simulink model "block6_simulink"  (R2025a)
settings: Solver=ode23tb  StartTime=0.0  StopTime=9  RelTol=1e-3
values from neighbouring files (symbols this model uses):
  K = inv(Rm) * B' * P    [block_6.m]
undefined symbols (not defined in the file or in its folder): G, I0_nom, iL_nom, Jac_A_lin, Jac_B_lin, R, V0, vC_nom
libraries: SignalEditorBlockLib x1
settings Model: Creator=arntzen  LastModifiedBy=arntzen

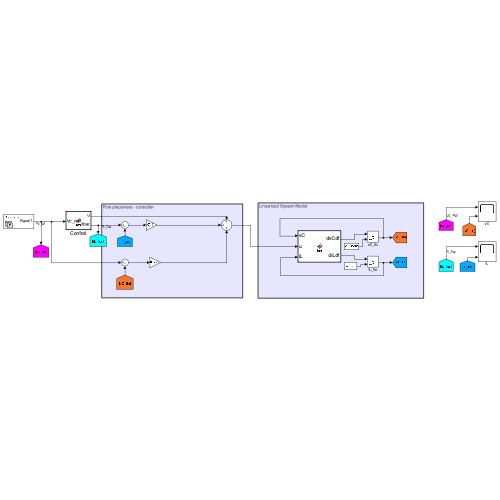
[thumbnail: Simulink's stored preview of the top-level diagram]
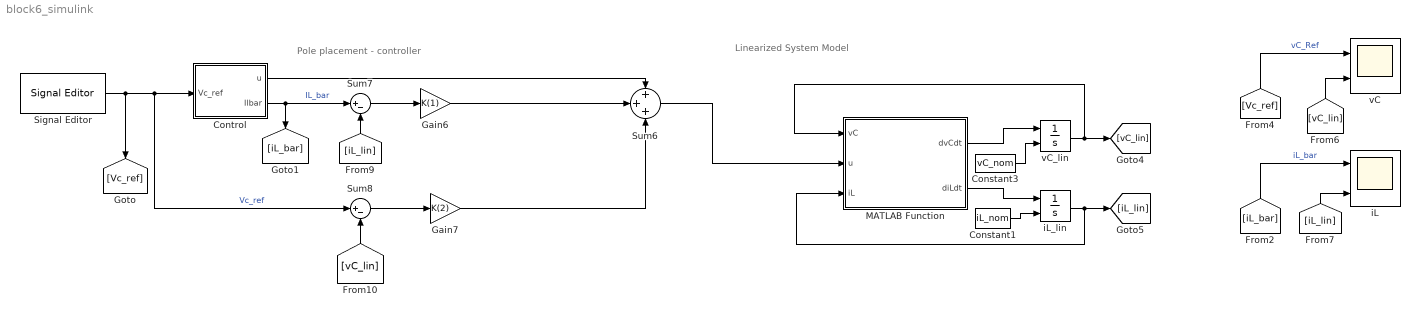
== system block6_simulink ==
  note: Pole placement - controller
  note: Linearized System Model
  Constant1 : Constant  Value=iL_nom
  Constant3 : Constant  Value=vC_nom
  Control : MATLAB Function  TreatAsAtomicUnit=on
  Gain6 : Gain  Gain=K(1)
  Gain7 : Gain  Gain=K(2)
  MATLAB Function : MATLAB Function  TreatAsAtomicUnit=on
  Signal Editor : SignalEditorBlockLib/Signal Editor  FileName=Block_6_signaleditor.mat  ActiveScenario=Scenario  ActiveSignal=Signal 1  IsBus=off  OutputBusObjectStr=Bus: BusObject  SampleTime=0  ZeroCross=off  OutputAfterFinalValue=Setting to zero  Unit=inherit  PreserveSignalName=on  ApplySigPropsToAllScenarios=on  ApplySigPropsToAllSignals=off  SignalPropertySource=Dialog parameters
  Sum6 : Sum  Inputs=+++
  Sum7 : Sum  Inputs=|+-
  Sum8 : Sum  Inputs=|+-
  iL : Scope  NumInputPorts=2
      settings: ActiveDisplayYMinimum=2.9172908696082791  ActiveDisplayYMaximum=10.140957946484352
  iL_lin : Integrator  InitialConditionSource=external
  vC : Scope  NumInputPorts=2
      settings: ActiveDisplayYMinimum=6.1422127164470979  ActiveDisplayYMaximum=24.720085551976119
  vC_lin : Integrator  InitialConditionSource=external
  wires:
  Signal Editor/1 -> [Vc_ref], Sum8/1, Control/1(Vc_ref)  "Vc_ref"
  MATLAB Function/1(dvCdt) -> vC_lin/1
  MATLAB Function/2(diLdt) -> iL_lin/1
  vC_lin/1 -> MATLAB Function/1(vC), [vC_lin]
  iL_lin/1 -> [iL_lin], MATLAB Function/3(iL)
  [iL_bar] -> iL/1  "iL_bar"
  [Vc_ref] -> vC/1  "vC_Ref"
  Constant3/1 -> vC_lin/2
  Constant1/1 -> iL_lin/2
  [vC_lin] -> vC/2
  [iL_lin] -> iL/2
  [iL_lin] -> Sum7/2
  [vC_lin] -> Sum8/2
  Sum8/1 -> Gain7/1
  Sum7/1 -> Gain6/1
  Sum6/1 -> MATLAB Function/2(u)
  Control/2(Ilbar) -> [iL_bar], Sum7/1  "IL_bar"
  Gain6/1 -> Sum6/2
  Gain7/1 -> Sum6/3
  Control/1(u) -> Sum6/1

== matlab function block6_simulink/Control ==
  data: u output; V0 parameter; R parameter; G parameter; I0_nom parameter; Vc_ref input; Ilbar output
function [u, Ilbar] = fcn(V0, R, G, I0_nom, Vc_ref)

Ilbar = (V0 - sqrt(V0^2 - 4*R*(G*Vc_ref^2 + I0_nom*Vc_ref))) / (2*R);
u = 1 - (G*Vc_ref + I0_nom) / Ilbar

== matlab function block6_simulink/MATLAB Function ==
  data: vC input; u input; iL input; dvCdt output; Jac_A_lin parameter; Jac_B_lin parameter; E parameter; diLdt output
function [dvCdt, diLdt]  = fcn(vC, u, iL, Jac_A_lin, Jac_B_lin, E)

x = [iL
     vC]

dxdt = Jac_A_lin * x + Jac_B_lin * u + E;

diLdt = dxdt(1);
dvCdt = dxdt(2);
